simulink model "ControlloAdattativo"  (R2021a)
settings: Solver=VariableStepAuto  StartTime=0.0  StopTime=50  RelTol=1e-3
values from neighbouring files (symbols this model uses):
  KD = kdi*eye(4)    [traiettoria.m]
  Kd = 200*diag([1 1 1 1])    [traiettoria.m]
  KP = kpi*eye(4)    [traiettoria.m]
  LAMBDA = 500*diag([1 1 1 1])    [traiettoria.m]
  q0 = scara.ikine(T0, 'mask', [1 1 1 1 0 0])    [pseudo_traiettoria.m]    (also in traiettoria.m)
  Tc = 0.001    [pseudo_traiettoria.m]    (also in traiettoria.m)
undefined symbols (not defined in the file or in its folder): DiscIntNeverNeededParam
settings Model: Creator=Ciro  LastModifiedBy=Ciro

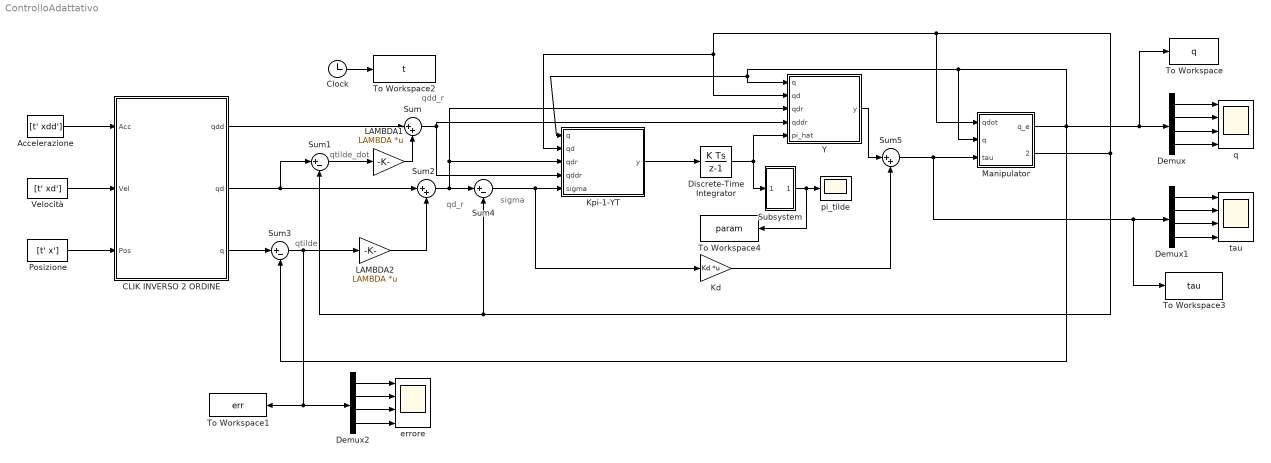
== system ControlloAdattativo ==
  note: qd_r
  note: qtilde_dot
  note: qtilde
  note: sigma
  note: qdd_r
  Accelerazione : FromWorkspace  VariableName=[t' xdd']  SampleTime=Tc  OutputAfterFinalValue=Holding final value
  CLIK INVERSO 2 ORDINE : Subsystem
  Clock : Clock
  Demux : Demux
  Demux1 : Demux
  Demux2 : Demux
  Discrete-Time Integrator : DiscreteIntegrator  InitialCondition=[25; 5; 0.02; 0.0001; 25; 5; 0.02; 0.0001; 10; 0.005; 0.01; 1; 0.001; 0.005]  SampleTime=-1  ICPrevOutput=DiscIntNeverNeededParam  ICPrevScaledInput=DiscIntNeverNeededParam
  Kd : Gain  Gain=Kd  Multiplication=Matrix(K*u)
  Kpi-1-YT : MATLAB Function  TreatAsAtomicUnit=on
  LAMBDA1 : Gain  Gain=LAMBDA  Multiplication=Matrix(K*u)
  LAMBDA2 : Gain  Gain=LAMBDA  Multiplication=Matrix(K*u)
  Manipulator : Subsystem
  Posizione : FromWorkspace  VariableName=[t' x']  SampleTime=Tc  OutputAfterFinalValue=Holding final value
  Subsystem : Subsystem
  Sum : Sum  Inputs=|++
  Sum1 : Sum  Inputs=|+-
  Sum2 : Sum  Inputs=|++
  Sum3 : Sum  Inputs=|+-
  Sum4 : Sum  Inputs=|+-
  Sum5 : Sum  Inputs=|++
  To Workspace : ToWorkspace  VariableName=q  SampleTime=-1
      settings: Save2DSignal=2-D array (concatenate along first dimension)
  To Workspace1 : ToWorkspace  VariableName=err  SampleTime=-1
      settings: Save2DSignal=2-D array (concatenate along first dimension)
  To Workspace2 : ToWorkspace  VariableName=t  SampleTime=-1
      settings: Save2DSignal=2-D array (concatenate along first dimension)
  To Workspace3 : ToWorkspace  VariableName=tau  SampleTime=-1
      settings: Save2DSignal=2-D array (concatenate along first dimension)
  To Workspace4 : ToWorkspace  VariableName=param  SampleTime=-1
      settings: Save2DSignal=2-D array (concatenate along first dimension)
  Velocità : FromWorkspace  VariableName=[t' xd']  SampleTime=Tc  OutputAfterFinalValue=Holding final value
  Y : MATLAB Function  TreatAsAtomicUnit=on
  errore : Scope  NumInputPorts=4
  pi_tilde : Scope
  q : Scope  NumInputPorts=4
  tau : Scope  NumInputPorts=4
  wires:
  Posizione/1 -> CLIK INVERSO 2 ORDINE/3(Pos)
  Velocità/1 -> CLIK INVERSO 2 ORDINE/2(Vel)
  Accelerazione/1 -> CLIK INVERSO 2 ORDINE/1(Acc)
  CLIK INVERSO 2 ORDINE/1(qdd) -> Sum/1
  Sum1/1 -> LAMBDA1/1
  LAMBDA1/1 -> Sum/2
  CLIK INVERSO 2 ORDINE/2(qd) -> Sum1/1, Sum2/1
  CLIK INVERSO 2 ORDINE/3(q) -> Sum3/1
  LAMBDA2/1 -> Sum2/2
  Sum2/1 -> Y/3(qdr), Kpi-1-YT/3(qdr), Sum4/1
  Sum4/1 -> Kd/1, Kpi-1-YT/5(sigma)
  Kpi-1-YT/1(y) -> Discrete-Time Integrator/1
  Discrete-Time Integrator/1 -> Subsystem/1(In1), Y/5(pi_hat)
  Y/1(y) -> Sum5/1
  Kd/1 -> Sum5/2
  Manipulator/1(q_e) -> Sum3/2, To Workspace/1, Demux/1, Manipulator/2(q), Y/1(q), Kpi-1-YT/1(q)
  Manipulator/2(qdot_e) -> Sum1/2, Sum4/2, Manipulator/1(qdot), Y/2(qd), Kpi-1-YT/2(qd)
  Sum/1 -> Y/4(qddr), Kpi-1-YT/4(qddr)
  Demux/1 -> q/1
  Demux/3 -> q/3
  Demux/2 -> q/2
  Demux/4 -> q/4
  Demux1/4 -> tau/4
  Demux1/2 -> tau/2
  Demux1/3 -> tau/3
  Demux1/1 -> tau/1
  Sum3/1 -> Demux2/1, To Workspace1/1, LAMBDA2/1
  Demux2/1 -> errore/1
  Demux2/3 -> errore/3
  Demux2/2 -> errore/2
  Demux2/4 -> errore/4
  Clock/1 -> To Workspace2/1
  Sum5/1 -> To Workspace3/1, Demux1/1, Manipulator/3(tau)
  Subsystem/1(Out1) -> To Workspace4/1, pi_tilde/1

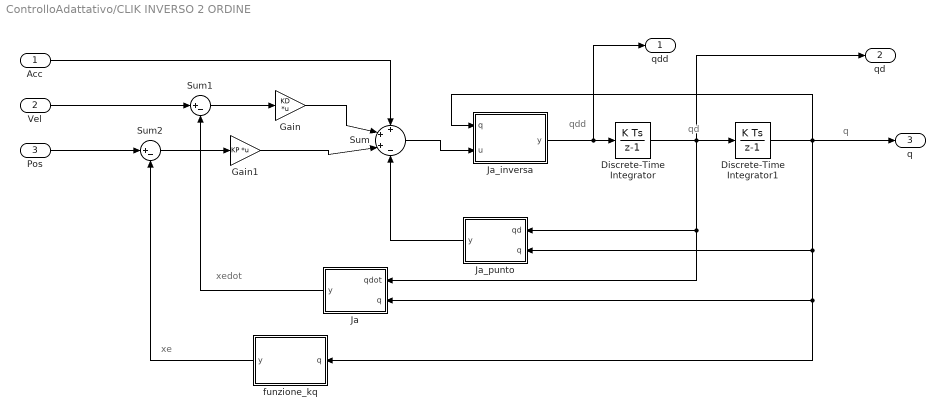
== system ControlloAdattativo/CLIK INVERSO 2 ORDINE ==
  note: qdd
  note: xedot
  note: xe
  note: qd
  note: q
  Acc : Inport
  Vel : Inport  Port=2
  Pos : Inport  Port=3
  Discrete-Time Integrator : DiscreteIntegrator  InitialCondition=[0; 0; 0; 0]  SampleTime=Tc  ICPrevOutput=DiscIntNeverNeededParam  ICPrevScaledInput=DiscIntNeverNeededParam
  Discrete-Time Integrator1 : DiscreteIntegrator  InitialCondition=q0  SampleTime=Tc  ICPrevOutput=DiscIntNeverNeededParam  ICPrevScaledInput=DiscIntNeverNeededParam
  Gain : Gain  Gain=KD  Multiplication=Matrix(K*u)
  Gain1 : Gain  Gain=KP  Multiplication=Matrix(K*u)
  Ja : MATLAB Function  TreatAsAtomicUnit=on
  Ja_inversa : MATLAB Function  TreatAsAtomicUnit=on
  Ja_punto : MATLAB Function  TreatAsAtomicUnit=on
  Sum : Sum  Inputs=+++-
  Sum1 : Sum  Inputs=|+-
  Sum2 : Sum  Inputs=|+-
  funzione_kq : MATLAB Function  TreatAsAtomicUnit=on
  qdd : Outport
  qd : Outport  Port=2
  q : Outport  Port=3
  wires:
  Gain1/1 -> Sum/3
  Discrete-Time Integrator1/1 -> q/1, Ja_punto/2(q), Ja/2(q), funzione_kq/1(q), Ja_inversa/1(q)
  Ja_punto/1(y) -> Sum/4
  Pos/1 -> Sum2/1
  Sum/1 -> Ja_inversa/2(u)
  Gain/1 -> Sum/2
  Sum2/1 -> Gain1/1
  funzione_kq/1(y) -> Sum2/2
  Ja/1(y) -> Sum1/2
  Sum1/1 -> Gain/1
  Vel/1 -> Sum1/1
  Acc/1 -> Sum/1
  Discrete-Time Integrator/1 -> qd/1, Ja_punto/1(qd), Ja/1(qdot), Discrete-Time Integrator1/1
  Ja_inversa/1(y) -> qdd/1, Discrete-Time Integrator/1

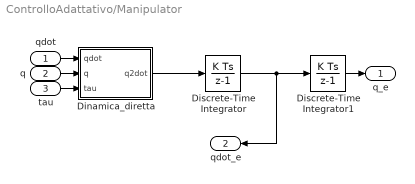
== system ControlloAdattativo/Manipulator ==
  qdot : Inport
  q : Inport  Port=2
  tau : Inport  Port=3
  Dinamica_diretta : MATLAB Function  TreatAsAtomicUnit=on
  Discrete-Time Integrator : DiscreteIntegrator  InitialCondition=[0; 0; 0; 0]  SampleTime=Tc  ICPrevOutput=DiscIntNeverNeededParam  ICPrevScaledInput=DiscIntNeverNeededParam
  Discrete-Time Integrator1 : DiscreteIntegrator  InitialCondition=q0  SampleTime=Tc  ICPrevOutput=DiscIntNeverNeededParam  ICPrevScaledInput=DiscIntNeverNeededParam
  q_e : Outport
  qdot_e : Outport  Port=2
  wires:
  tau/1 -> Dinamica_diretta/3(tau)
  qdot/1 -> Dinamica_diretta/1(qdot)
  q/1 -> Dinamica_diretta/2(q)
  Discrete-Time Integrator1/1 -> q_e/1
  Discrete-Time Integrator/1 -> Discrete-Time Integrator1/1, qdot_e/1
  Dinamica_diretta/1(q2dot) -> Discrete-Time Integrator/1

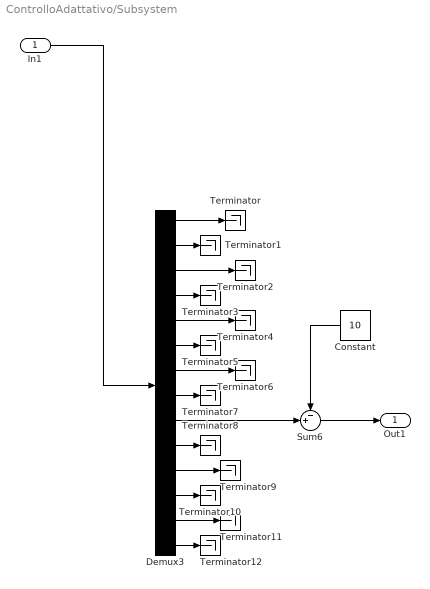
== system ControlloAdattativo/Subsystem ==
  In1 : Inport
  Constant : Constant  Value=10
  Demux3 : Demux  Outputs=14
  Sum6 : Sum  Inputs=-+|
  Terminator{,1..12} (13 alike) : Terminator
  Out1 : Outport
  wires:
  Demux3/12 -> Terminator10/1
  Demux3/9 -> Sum6/2
  Demux3/6 -> Terminator5/1
  In1/1 -> Demux3/1
  Demux3/1 -> Terminator/1
  Demux3/2 -> Terminator1/1
  Demux3/14 -> Terminator12/1
  Demux3/11 -> Terminator9/1
  Constant/1 -> Sum6/1
  Demux3/10 -> Terminator8/1
  Demux3/5 -> Terminator4/1
  Demux3/3 -> Terminator2/1
  Demux3/4 -> Terminator3/1
  Demux3/13 -> Terminator11/1
  Demux3/8 -> Terminator7/1
  Demux3/7 -> Terminator6/1
  Sum6/1 -> Out1/1

== matlab function ControlloAdattativo/CLIK INVERSO 2 ORDINE/funzione_kq ==
  data: q input; y output
function y = fcn(q)

xe = [0.5*(cos(q(1))+cos(q(1)+q(2)));
      0.5*(sin(q(1))+sin(q(1)+q(2)));
      0.8-q(3);
      q(1)+q(2)-q(4)];

y = xe;

== matlab function ControlloAdattativo/CLIK INVERSO 2 ORDINE/Ja_inversa ==
  data: q input; u input; y output
function y = fcn(q, u)
J = [ -0.5*(sin(q(1))+sin(q(1)+q(2))) -0.5*sin(q(1)+q(2))  0  0;
       0.5*(cos(q(1))+cos(q(1)+q(2)))  0.5*cos(q(1)+q(2))  0  0;
       0                               0                  -1  0;
       1                               1                   0 -1];
y = inv(J)*u;

== matlab function ControlloAdattativo/CLIK INVERSO 2 ORDINE/Ja ==
  data: qdot input; q input; y output
function y = fcn(qdot,q)
J = [ -0.5*(sin(q(1))+sin(q(1)+q(2))) -0.5*sin(q(1)+q(2))  0  0;
       0.5*(cos(q(1))+cos(q(1)+q(2)))  0.5*cos(q(1)+q(2))  0  0;
       0                               0                  -1  0;
       1                               1                   0 -1];
y = J*qdot;

== matlab function ControlloAdattativo/CLIK INVERSO 2 ORDINE/Ja_punto ==
  data: qd input; q input; y output
function y = fcn(qd,q)
Jpunto = [ -0.5*(cos(q(1))*qd(1) + cos(q(1)+q(2))*(qd(1)+qd(2)))    -0.5*cos(q(1)+q(2))*(qd(1)+qd(2))  0  0;
           -0.5*(sin(q(1))*qd(1) + sin(q(1)+q(2))*(qd(1)+qd(2)))    -0.5*sin(q(1)+q(2))*(qd(1)+qd(2))  0  0;
           0                                                        0                                  0  0;
           0                                                        0                                  0  0];
y = Jpunto*qd;

== matlab function ControlloAdattativo/Kpi-1-YT ==
  data: q input; qd input; qdr input; qddr input; sigma input; y output
function y = fcn(q,qd,qdr,qddr,sigma)

%rapporti di trasmissione;
Kr1 = 1;
Kr2 = 1;
Kr3 = 50;
Kr4 = 20;

L1 = 0.25;
L2 = 0.25;

a1 = 0.5;
a2 = 0.5;

Y = zeros(4,14);
q1 = q(1);
q2 = q(2);
q3 = q(3);
q4 = q(4);
q1d = qd(1);
q2d = qd(2);
q3d = qd(3);
q4d = qd(4);
q1dr = qdr(1);
q2dr = qdr(2);
q3dr = qdr(3);
q4dr = qdr(4);
q1ddr = qddr(1);
q2ddr = qddr(2);
q3ddr = qddr(3);
q4ddr = qddr(4);

Y(1,1) = q1ddr*L1^2;
Y(1,2) = q1ddr;
Y(1,3) = q1ddr*Kr1^2;
Y(1,4) = -q1dr*Kr1^2;
Y(1,5) = (q1ddr+q2ddr)*L2^2+q1ddr*a1^2+ 2*L2*a1*q1ddr*cos(q2) + L2*a1*q2ddr*cos(q2) - L2*a1*q1d*q2dr*sin(q2) - L2*a1*q2d*q1dr*sin(q2) - L2*a1*q2d*q2dr*sin(q2);
Y(1,6) = q1ddr+q2ddr;
Y(1,7) = q1ddr;
Y(1,8) = 0;
Y(1,9) = (a1^2+a2^2)*q1ddr + q2ddr*a2^2 + 2*a1*a2*q1ddr*cos(q2) + a1*a2*q2ddr*cos(q2)-a1*a2*q1d*q2dr*sin(q2)-a1*a2*q2d*q1dr*sin(q2)-a1*a2*q2d*q2dr*sin(q2);
Y(1,10) = q1ddr+q2ddr;
Y(1,11) = 0;
Y(1,12) = q1ddr+q2ddr-q4ddr;
Y(1,13) = q1ddr+q2ddr-q4ddr;
Y(1,14) = 0;

Y(2,1) = 0;
Y(2,2) = 0;
Y(2,3) = 0;
Y(2,4) = 0;
Y(2,5) = (q1ddr+q2ddr)*L2^2 + L2*a1*q1ddr*cos(q2) + L2*a1*q1d*q1dr*sin(q2);
Y(2,6) = q1ddr+q2ddr;
Y(2,7) = q2ddr*Kr2^2;
Y(2,8) = -q2dr*Kr2^2;
Y(2,9) = (q2ddr+q1ddr)*a2^2 + a1*a2*q1ddr*cos(q2) + a1*a2*q1d*q1dr*sin(q2);
Y(2,10) = q1ddr+q2ddr;
Y(2,11) = 0;
Y(2,12) = q1ddr+q2ddr-q4ddr;
Y(2,13) = q1ddr+q2ddr-q4ddr;
Y(2,14) = 0;

Y(3,1) = 0;
Y(3,2) = 0;
Y(3,3) = 0;
Y(3,4) = 0;
Y(3,5) = 0;
Y(3,6) = 0;
Y(3,7) = 0;
Y(3,8) = 0;
Y(3,9) = q3ddr-9.81;
Y(3,10) = q3ddr*Kr3^2;
Y(3,11) = -q3dr*Kr3^2;
Y(3,12) = 0;
Y(3,13) = 0;
Y(3,14) = 0;

Y(4,1) = 0;
Y(4,2) = 0;
Y(4,3) = 0;
Y(4,4) = 0;
Y(4,5) = 0;
Y(4,6) = 0;
Y(4,7) = 0;
Y(4,8) = 0;
Y(4,9) = 0;
Y(4,10) = 0;
Y(4,11) = 0;
Y(4,12) = q4ddr-q2ddr-q1ddr;
Y(4,13) = q4ddr-q2ddr-q1ddr+q4ddr*Kr4^2;
Y(4,14) = -q4dr*Kr4^2;

K = 10000;
Kpi = K*diag([1 1 1 1 1 1 1 1 2/K 1 1 1 1 1]);

y = inv(Kpi)*(Y')*sigma;

== matlab function ControlloAdattativo/Y ==
  data: q input; qd input; qdr input; qddr input; pi_hat input; y output
function y = fcn(q,qd,qdr,qddr,pi_hat)

Kr1 = 1;
Kr2 = 1;
Kr3 = 50;
Kr4 = 20;

L1 = 0.25;
L2 = 0.25;

a1 = 0.5;
a2 = 0.5;

Y = zeros(4,14);
q1 = q(1);
q2 = q(2);
q3 = q(3);
q4 = q(4);
q1d = qd(1);
q2d = qd(2);
q3d = qd(3);
q4d = qd(4);
q1dr = qdr(1);
q2dr = qdr(2);
q3dr = qdr(3);
q4dr = qdr(4);
q1ddr = qddr(1);
q2ddr = qddr(2);
q3ddr = qddr(3);
q4ddr = qddr(4);

Y(1,1) = q1ddr*L1^2;
Y(1,2) = q1ddr;
Y(1,3) = q1ddr*Kr1^2;
Y(1,4) = -q1dr*Kr1^2;
Y(1,5) = (q1ddr+q2ddr)*L2^2+q1ddr*a1^2+ 2*L2*a1*q1ddr*cos(q2) + L2*a1*q2ddr*cos(q2) - L2*a1*q1d*q2dr*sin(q2) - L2*a1*q2d*q1dr*sin(q2) - L2*a1*q2d*q2dr*sin(q2);
Y(1,6) = q1ddr+q2ddr;
Y(1,7) = q1ddr;
Y(1,8) = 0;
Y(1,9) = (a1^2+a2^2)*q1ddr + q2ddr*a2^2 + 2*a1*a2*q1ddr*cos(q2) + a1*a2*q2ddr*cos(q2)-a1*a2*q1d*q2dr*sin(q2)-a1*a2*q2d*q1dr*sin(q2)-a1*a2*q2d*q2dr*sin(q2);
Y(1,10) = q1ddr+q2ddr;
Y(1,11) = 0;
Y(1,12) = q1ddr+q2ddr-q4ddr;
Y(1,13) = q1ddr+q2ddr-q4ddr;
Y(1,14) = 0;

Y(2,1) = 0;
Y(2,2) = 0;
Y(2,3) = 0;
Y(2,4) = 0;
Y(2,5) = (q1ddr+q2ddr)*L2^2 + L2*a1*q1ddr*cos(q2) + L2*a1*q1d*q1dr*sin(q2);
Y(2,6) = q1ddr+q2ddr;
Y(2,7) = q2ddr*Kr2^2;
Y(2,8) = -q2dr*Kr2^2;
Y(2,9) = (q2ddr+q1ddr)*a2^2 + a1*a2*q1ddr*cos(q2) + a1*a2*q1d*q1dr*sin(q2);
Y(2,10) = q1ddr+q2ddr;
Y(2,11) = 0;
Y(2,12) = q1ddr+q2ddr-q4ddr;
Y(2,13) = q1ddr+q2ddr-q4ddr;
Y(2,14) = 0;

Y(3,1) = 0;
Y(3,2) = 0;
Y(3,3) = 0;
Y(3,4) = 0;
Y(3,5) = 0;
Y(3,6) = 0;
Y(3,7) = 0;
Y(3,8) = 0;
Y(3,9) = q3ddr-9.81;
Y(3,10) = q3ddr*Kr3^2;
Y(3,11) = -q3dr*Kr3^2;
Y(3,12) = 0;
Y(3,13) = 0;
Y(3,14) = 0;

Y(4,1) = 0;
Y(4,2) = 0;
Y(4,3) = 0;
Y(4,4) = 0;
Y(4,5) = 0;
Y(4,6) = 0;
Y(4,7) = 0;
Y(4,8) = 0;
Y(4,9) = 0;
Y(4,10) = 0;
Y(4,11) = 0;
Y(4,12) = q4ddr-q2ddr-q1ddr;
Y(4,13) = q4ddr-q2ddr-q1ddr+q4ddr*Kr4^2;
Y(4,14) = -q4dr*Kr4^2;

y = Y*pi_hat;

== matlab function ControlloAdattativo/Manipulator/Dinamica_diretta ==
  data: qdot input; q input; tau input; q2dot output
function q2dot = fcn(qdot,q,tau)

a1 = 0.5;
a2 = 0.5;

%% Dinamica

%masse
ml1 = 25;
ml2 = 25;
ml3 = 10;

%posizioni baricentro
L1 = 0.25;
L2 = 0.25;

%inerzie di massa bracci
Il1 = 5;
Il2 = 5;
Il4 = 1;

%rapporti di trasmissione;
Kr1 = 1;
Kr2 = 1;
Kr3 = 50;
Kr4 = 20;

%inerzie motori
Im1 = 0.02;
Im2 = 0.02;
Im3 = 0.005;
Im4 = 0.001;

%attriti dei motori
Fm1 = 0.0001;
Fm2 = 0.0001;
Fm3 = 0.01;
Fm4 = 0.005;

load = 5;

q2 = q(2);
q1d = qdot(1);
q2d = qdot(2);
q3d = qdot(3);
q4d = qdot(4);

B=[Il1 + Il2 + Il4 + Im2 + Im3 + Im4 + Im1*Kr1^2 + L1^2*ml1 + L2^2*ml2 + a1^2*load + a2^2*load + a1^2*ml2 + a1^2*ml3 + a2^2*ml3 + 2*L2*a1*ml2*cos(q2) + 2*a1*a2*load*cos(q2) + 2*a1*a2*ml3*cos(q2), Il2 + Il4 + Im3 + Im4 + L2^2*ml2 + a2^2*load + a2^2*ml3 + L2*a1*ml2*cos(q2) + a1*a2*load*cos(q2) + a1*a2*ml3*cos(q2),                      0,        - Il4 - Im4;
                                                                           Il2 + Il4 + Im3 + Im4 + L2^2*ml2 + a2^2*load + a2^2*ml3 + L2*a1*ml2*cos(q2) + a1*a2*load*cos(q2) + a1*a2*ml3*cos(q2),                                                  Il2 + Il4 + Im3 + Im4 + Im2*Kr2^2 + L2^2*ml2 + a2^2*load + a2^2*ml3,                      0,           - Il4 - Im4;
                                                                                                                                                                                              0,                                                                                                                    0, Im3*Kr3^2 + load + ml3,                     0;
                                                                                                                                                                                    - Il4 - Im4,                                                                                                          - Il4 - Im4,                      0, Im4*Kr4^2 + Il4 + Im4];
C = [-a1*q2d*sin(q2)*(L2*ml2 + a2*load + a2*ml3), -a1*sin(q2)*(q1d + q2d)*(L2*ml2 + a2*load + a2*ml3), 0, 0;
 a1*q1d*sin(q2)*(L2*ml2 + a2*load + a2*ml3),                                                   0, 0, 0;
                                          0,                                                   0, 0, 0;
                                          0,                                                   0, 0, 0];


Fv = [-Fm1*q1d*abs(Kr1)^2; -Fm2*q2d*abs(Kr2)^2; -Fm3*q3d*abs(Kr3)^2; -Fm4*q4d*abs(Kr4)^2];
g = [0, 0, - 9.81*load - 9.81*ml3, 0]';
tau_primo = C*qdot+Fv+g;

q2dot = inv(B)*(tau-tau_primo);
